simulink model "finger_mus2_20042021"  (R2020b)
settings: Solver=ode113  StartTime=0.0  StopTime=T  FixedStep=0.0001  RelTol=1e-4  EnableMultiTasking=on
values from neighbouring files (symbols this model uses):
  q1dot0 = 0    [settings2.mat]
  q1init = q10; clear q10    [hand_test.m]
  q2dot0 = 0    [settings2.mat]
  q2init = q20; clear q20    [hand_test.m]
  q3dot0 = 0    [settings2.mat]
  q3init = q30; clear q30    [hand_test.m]
  Ts = 0.02    [hand_test.m]
libraries: simulink x3
settings Model: Creator=djfh09v  LastModifiedBy=olivergrainge
settings DataIOCC: LimitDataPoints=on  SaveFormat=Array  SignalLoggingSaveFormat=ModelDataLogs  ReturnWorkspaceOutputs=off
settings OptimizationCC: ExpressionDepthLimit=2147483647  InitFltsAndDblsToZero=on  LifeSpan=inf
settings DebuggingCC: SaveWithParameterizedLinksMsg=none  UnderspecifiedInitializationDetection=Classic  MergeDetectMultiDrivingBlocksExec=none  SignalResolutionControl=TryResolveAllWithWarning  SolverPrmCheckMsg=warning  FcnCallInpInsideContextMsg=warning  StateNameClashWarn=warning  SFUnexpectedBacktrackingDiag=warning  SFNoUnconditionalDefaultTransitionDiag=warning  SFExecutionAtInitializationDiag=none  ArithmeticOperatorsInVariantConditions=warning
settings HardwareCC: ProdBitPerPointer=32  ProdBitPerSizeT=32  ProdBitPerPtrDiffT=32  ProdLargestAtomicFloat=None  ProdIntDivRoundTo=Undefined  ProdEndianess=Unspecified  ProdWordSize=32  ProdHWDeviceType=32-bit Generic
settings ModelReferenceCC: PropagateSignalLabelsOutOfModel=off
settings SFSimCC: SimUseLocalCustomCode=off  SimParseCustomCode=off  CustomCodeUndefinedFunction=UseInterfaceOnly
settings RTWCC: RTWUseLocalCustomCode=off
settings CodeAppCC: StateflowObjectComments=on
settings GRTTargetCC: TargetFcnLib=ansi_tfl_tmw.mat  TargetLangStandard=C89/C90 (ANSI)  CombineOutputUpdateFcns=off  GRTInterface=on
settings ConfigComp: CovMetricSettings=dw  CovSaveCumulativeToWorkspaceVar=on  CovSaveSingleToWorkspaceVar=on

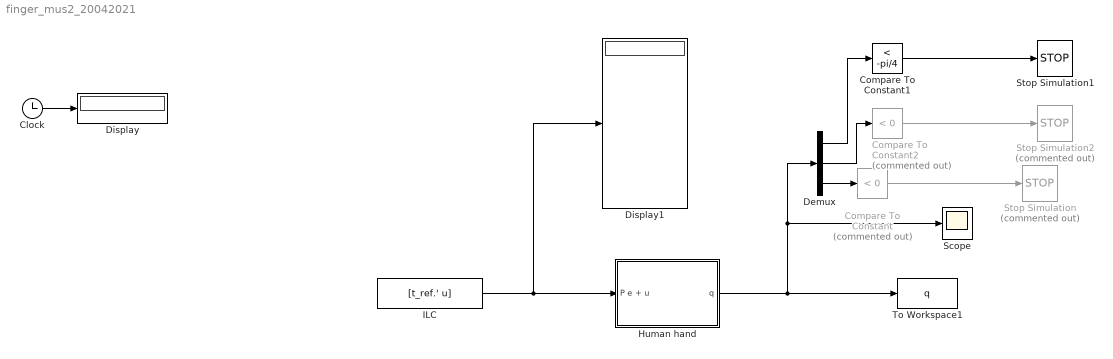
== system finger_mus2_20042021 ==
  Clock : Clock
  Compare To Constant : simulink/Logic and Bit Operations/Compare To Constant  Commented=on  relop=<  const=0  OutDataTypeStr=boolean
  Compare To Constant1 : simulink/Logic and Bit Operations/Compare To Constant  relop=<  const=-pi/4  OutDataTypeStr=boolean
  Compare To Constant2 : simulink/Logic and Bit Operations/Compare To Constant  Commented=on  relop=<  const=0  OutDataTypeStr=boolean
  Demux : Demux  Outputs=3
  Display : Display
  Display1 : Display
  Human hand : Subsystem
  ILC : FromWorkspace  VariableName=[t_ref.' u]
  Scope : Scope
  Stop Simulation : Stop  Commented=on
  Stop Simulation1 : Stop
  Stop Simulation2 : Stop  Commented=on
  To Workspace1 : ToWorkspace  VariableName=q  SaveFormat=Structure With Time  SampleTime=Ts
  wires:
  Clock/1 -> Display/1
  Human hand/1(q) -> To Workspace1/1, Scope/1, Demux/1
  ILC/1 -> Display1/1, Human hand/1(" P e + u")
  Demux/3 -> Compare To Constant/1
  Compare To Constant/1 -> Stop Simulation/1
  Compare To Constant1/1 -> Stop Simulation1/1
  Demux/1 -> Compare To Constant1/1
  Compare To Constant2/1 -> Stop Simulation2/1
  Demux/2 -> Compare To Constant2/1

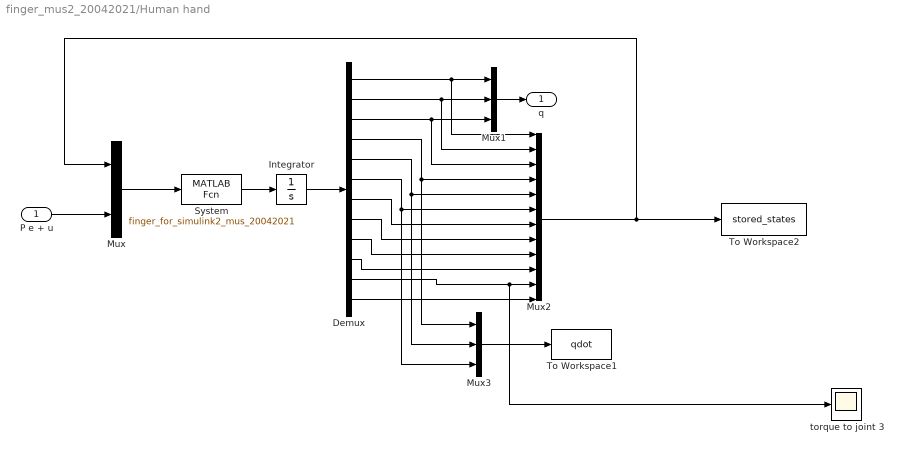
== system finger_mus2_20042021/Human hand ==
  " P e + u" : Inport
  Demux : Demux  Outputs=12
  Integrator : Integrator  InitialCondition="[q1init q2init q3init q1dot0 q2dot0 q3dot0  0  0  0  0  0  0]"
  Mux : Mux  Inputs=2
  Mux1 : Mux  Inputs=3
  Mux2 : Mux  Inputs=12
  Mux3 : Mux  Inputs=3
  System : MATLABFcn  MATLABFcn=finger_for_simulink2_mus_20042021  OutputDimensions=12
  To Workspace1 : ToWorkspace  VariableName=qdot  SaveFormat=Structure With Time  SampleTime=Ts
  To Workspace2 : ToWorkspace  VariableName=stored_states  SaveFormat=Structure With Time  SampleTime=Ts
  torque to joint 3 : Scope
  q : Outport
  wires:
  System/1 -> Integrator/1
  Mux/1 -> System/1
  Integrator/1 -> Demux/1
  Demux/1 -> Mux1/1, Mux2/1
  Demux/2 -> Mux1/2, Mux2/2
  Demux/3 -> Mux1/3, Mux2/3
  Mux1/1 -> q/1
  Mux2/1 -> Mux/1, To Workspace2/1
  Demux/4 -> Mux2/4, Mux3/1
  Mux3/1 -> To Workspace1/1
  " P e + u"/1 -> Mux/2
  Demux/5 -> Mux2/5, Mux3/2
  Demux/6 -> Mux2/6, Mux3/3
  Demux/7 -> Mux2/7
  Demux/8 -> Mux2/8
  Demux/9 -> Mux2/9
  Demux/10 -> Mux2/10
  Demux/11 -> torque to joint 3/1, Mux2/11
  Demux/12 -> Mux2/12
